simulink model "trim_homework태원"  (R2023b)
settings: Solver=VariableStepAuto  StartTime=0.0  StopTime=200  RelTol=1e-3
model workspace (MAT data in the model file):
  op_trim1 = opcond.OperatingReport
  op_trim1.Outputs_ = opcond.OutputReport
  op_trim1.Outputs_.yspec_ = 23
  op_trim1.Outputs_.Block_ = 'trim_homework/Va'
  op_trim1.Outputs_.PortWidth_ = 1
  op_trim1.Outputs_.PortNumber_ = NaN
  op_trim1.Outputs_.y_ = 23
  op_trim1.Outputs_.Known_ = 1
  op_trim1.Outputs_.Min_ = -Inf
  op_trim1.Outputs_.Max_ = Inf
  op_trim1.TerminationString_ = '동작점 사양이 성공적으로 충족되었습니다.'
  op_trim1.OptimizationOutput_.iterations = 4
  op_trim1.OptimizationOutput_.funcCount = 67
  op_trim1.OptimizationOutput_.lssteplength = 1
  op_trim1.OptimizationOutput_.stepsize = 1.37227351892e-10
  op_trim1.OptimizationOutput_.algorithm = 'active-set'
  op_trim1.OptimizationOutput_.firstorderopt = 0
  op_trim1.OptimizationOutput_.constrviolation = 8.72514182054e-12
  op_trim1.OptimizationOutput_.message = '제약 조건을 충족하는 국소 최솟값을 찾았습니다.
    | 
    | 목적 함수가 최적성 허용오차의 값 이내에서 실현 가능한 방향에서 감소하지 않고 
    | 제약 조건이 제약 조건 허용오차의 값 이내에서 충족되기 때문에 
    | 최적화가 완료되었습니다.
    | 
    | <중지 기준 세부 정보>
    | 
    | 최적화가 완료됨: 1차 최적성 측정값 0.000000e+00이(가)
    | options.OptimalityTolerance = 1.000000e-06보다 작고 최대 제약 조건 위반
    | 8.725142e-12이(가) options.ConstraintTolerance = 1.000000e-06보다 작습니다.'
  op_trim1.OptimizationOutput_.bestfeasible.x = [22.9488032673; 3.41196938771e-08; 1.53376288852; 1.51318063862e-09; 0.0667348663763; -1.38255798073e-09; 1.08686704389e-15; -3.74282177879e-15; 1.13331068217e-24; 4.09052789101e-22; 7.74880795459e-26; 1.11476618756e-09; -0.171064175627; 1.39174657063e-09; 11.2753696029]
  op_trim1.OptimizationOutput_.bestfeasible.fval = 0
  op_trim1.OptimizationOutput_.bestfeasible.constrviolation = 8.72514182054e-12
  op_trim1.OptimizationOutput_.bestfeasible.firstorderopt = 0
  op_trim1.OptimizationOutput_.progress = {'<font face="monospaced"; size=3><BR>', '원하는 dx/dt=0, x(k+1)-x(k)=0, y=ydes 전체에 대해 해를 구하기 위해 최적화합니다.<BR>', ' <BR>', '(최대 오차) 블록<BR>', ' ---------------------------------------------------------<BR>', '(5.95306e+00) trim_homework/6DOF (Euler Angles)/ub,vb,wb<BR>', '(3.93818e-01) trim_homework/6DOF (Euler Angles)/ub,vb,wb<BR>', '(2.71037e-05) trim_homework/6DOF (Euler Angles)/ub,vb,wb<BR>', '(8.72514e-12) trim_homework/6DOF (Euler Angles)/ub,vb,wb<BR>', '(8.72514e-12) trim_homework/6DOF (Euler Angles)/ub,vb,wb<BR>', ' <BR>', '동작점 사양이 성공적으로 충족되었습니다.<BR>'}
  op_trim1.Model_ = 'trim_homework'
  op_trim1.States_(1) = opcond.StateReport
  op_trim1.States_(1).dx_ = [1.13848957052e-24; 4.09052789101e-22; 7.76615688898e-26]
  op_trim1.States_(1).Nx_ = 3
  op_trim1.States_(1).Block_ = 'trim_homework/6DOF (Euler Angles)/Calculate DCM &
    | Euler Angles/phi
    | theta
    | psi'
  op_trim1.States_(1).x_ = [1.51318063862e-09; 0.0667348663763; -1.38255798073e-09]
  op_trim1.States_(1).SteadyState_ = [1; 1; 1]
  op_trim1.States_(1).dxMin_ = [-Inf; -Inf; -Inf]
  op_trim1.States_(1).dxMax_ = [Inf; Inf; Inf]
  op_trim1.States_(1).Known_ = [0; 0; 0]
  op_trim1.States_(1).Min_ = [-Inf; -Inf; -Inf]
  op_trim1.States_(1).Max_ = [Inf; Inf; Inf]
  op_trim1.States_(2) = opcond.StateReport
  op_trim1.States_(2).dx_ = [8.46060064603e-19; 3.2482900909e-13; -1.72544390739e-19]
  op_trim1.States_(2).Nx_ = 3
  op_trim1.States_(2).Block_ = 'trim_homework/6DOF (Euler Angles)/p,q,r '
  op_trim1.States_(2).x_ = [1.13331068217e-24; 4.09052789101e-22; 7.74880795459e-26]
  op_trim1.States_(2).SteadyState_ = [1; 1; 1]
  op_trim1.States_(2).dxMin_ = [-Inf; -Inf; -Inf]
  op_trim1.States_(2).dxMax_ = [Inf; Inf; Inf]
  op_trim1.States_(2).Known_ = [0; 0; 0]
  op_trim1.States_(2).Min_ = [-Inf; -Inf; -Inf]
  op_trim1.States_(2).Max_ = [Inf; Inf; Inf]
  op_trim1.States_(3) = opcond.StateReport
  op_trim1.States_(3).dx_ = [8.72514182054e-12; 4.3787508586e-19; -2.2478987429e-13]
  op_trim1.States_(3).Nx_ = 3
  op_trim1.States_(3).Block_ = 'trim_homework/6DOF (Euler Angles)/ub,vb,wb'
  op_trim1.States_(3).x_ = [22.9488032673; 3.41196938771e-08; 1.53376288852]
  op_trim1.States_(3).SteadyState_ = [1; 1; 1]
  op_trim1.States_(3).dxMin_ = [-Inf; -Inf; -Inf]
  op_trim1.States_(3).dxMax_ = [Inf; Inf; Inf]
  op_trim1.States_(3).Known_ = [0; 0; 0]
  op_trim1.States_(3).Min_ = [-Inf; -Inf; -Inf]
  op_trim1.States_(3).Max_ = [Inf; Inf; Inf]
  op_trim1.States_(4) = opcond.StateReport
  op_trim1.States_(4).dx_ = [23; 1.31654190371e-17; 4.10782519111e-14]
  op_trim1.States_(4).Nx_ = 3
  op_trim1.States_(4).Block_ = 'trim_homework/6DOF (Euler Angles)/xe,ye,ze'
  op_trim1.States_(4).x_ = [1.08686704389e-15; -3.74282177879e-15; -200]
  op_trim1.States_(4).SteadyState_ = [0; 1; 1]
  op_trim1.States_(4).dxMin_ = [-Inf; -Inf; -Inf]
  op_trim1.States_(4).dxMax_ = [Inf; Inf; Inf]
  op_trim1.States_(4).Known_ = [0; 0; 1]
  op_trim1.States_(4).Min_ = [-Inf; -Inf; -Inf]
  op_trim1.States_(4).Max_ = [Inf; Inf; Inf]
  op_trim1.Inputs_(1) = opcond.InputReport
  op_trim1.Inputs_(1).Block_ = 'trim_homework/AIL'
  op_trim1.Inputs_(1).PortWidth_ = 1
  op_trim1.Inputs_(1).PortDimensions_ = [1 1]
  op_trim1.Inputs_(1).u_ = 1.11476618756e-09
  op_trim1.Inputs_(1).Known_ = 0
  op_trim1.Inputs_(1).Min_ = -Inf
  op_trim1.Inputs_(1).Max_ = Inf
  op_trim1.Inputs_(2) = opcond.InputReport
  op_trim1.Inputs_(2).Block_ = 'trim_homework/ELE'
  op_trim1.Inputs_(2).PortWidth_ = 1
  op_trim1.Inputs_(2).PortDimensions_ = [1 1]
  op_trim1.Inputs_(2).u_ = -0.171064175627
  op_trim1.Inputs_(2).Known_ = 0
  op_trim1.Inputs_(2).Min_ = -Inf
  op_trim1.Inputs_(2).Max_ = Inf
  op_trim1.Inputs_(3) = opcond.InputReport
  op_trim1.Inputs_(3).Block_ = 'trim_homework/RUD'
  op_trim1.Inputs_(3).PortWidth_ = 1
  op_trim1.Inputs_(3).PortDimensions_ = [1 1]
  op_trim1.Inputs_(3).u_ = 1.39174657063e-09
  op_trim1.Inputs_(3).Known_ = 0
  op_trim1.Inputs_(3).Min_ = -Inf
  op_trim1.Inputs_(3).Max_ = Inf
  op_trim1.Inputs_(4) = opcond.InputReport
  op_trim1.Inputs_(4).Block_ = 'trim_homework/Thro'
  op_trim1.Inputs_(4).PortWidth_ = 1
  op_trim1.Inputs_(4).PortDimensions_ = [1 1]
  op_trim1.Inputs_(4).u_ = 11.2753696029
  op_trim1.Inputs_(4).Known_ = 0
  op_trim1.Inputs_(4).Min_ = -Inf
  op_trim1.Inputs_(4).Max_ = Inf
  op_trim2 = opcond.OperatingReport
  op_trim2.Outputs_ = opcond.OutputReport
  op_trim2.Outputs_.yspec_ = 23
  op_trim2.Outputs_.Block_ = 'trim_homework/Va'
  op_trim2.Outputs_.PortWidth_ = 1
  op_trim2.Outputs_.PortNumber_ = NaN
  op_trim2.Outputs_.y_ = 1
  op_trim2.Outputs_.Known_ = 1
  op_trim2.Outputs_.Min_ = -Inf
  op_trim2.Outputs_.Max_ = Inf
  op_trim2.TerminationString_ = '모든 제약 조건을 충족하는 해를 찾을 수 없습니다. 실현 가능한 해를 찾으려면 제약 조건을 완화하십시오.'
  op_trim2.OptimizationOutput_.iterations = 1
  op_trim2.OptimizationOutput_.funcCount = 25
  op_trim2.OptimizationOutput_.lssteplength = 1
  op_trim2.OptimizationOutput_.stepsize = 0
  op_trim2.OptimizationOutput_.algorithm = 'active-set'
  op_trim2.OptimizationOutput_.firstorderopt = []
  op_trim2.OptimizationOutput_.constrviolation = 22
  op_trim2.OptimizationOutput_.message = '실현불가능점으로 수렴되었습니다.
    | 
    | 현재 탐색 방향의 크기가 스텝 크기 허용오차 값의 두 배보다 
    | 작지만 제약 조건이 제약 조건 허용오차의 값 이내에서 
    | 충족되지 않기 때문에 fmincon이(가) 중지되었습니다.
    | 
    | <중지 기준 세부 정보>
    | 
    | 현재 탐색 방향의 노름 0.000000e+00이(가) 2*options.StepTolerance = 1.000000e-06보다
    | 작지만 최대 제약 조건 위반 2.200000e+01이(가) options.ConstraintTolerance = 1.000000e-06을(를)
    | 초과하기 때문에 최적화가 중지되었습니다.'
  op_trim2.OptimizationOutput_.bestfeasible = []
  op_trim2.OptimizationOutput_.progress = {'<font face="monospaced"; size=3><BR>', '원하는 dx/dt=0, x(k+1)-x(k)=0, y=ydes 전체에 대해 해를 구하기 위해 최적화합니다.<BR>', ' <BR>', '(최대 오차) 블록<BR>', ' ---------------------------------------------------------<BR>', '(2.20000e+01) trim_homework/Va<BR>', '(2.20000e+01) trim_homework/Va<BR>', ' <BR>', '모든 제약 조건을 충족하는 해를 찾을 수 없습니다. 실현 가능한 해를 찾으려면 제약 조건을 완화하십시오.<BR>'}
  op_trim2.Model_ = 'trim_homework'
  op_trim2.States_(1) = opcond.StateReport
  op_trim2.States_(1).dx_ = [0; 0; 0]
  op_trim2.States_(1).Nx_ = 3
  op_trim2.States_(1).Block_ = 'trim_homework/6DOF (Quaternion)/Calculate DCM &
    | Euler Angles/phi
    | theta
    | psi'
  op_trim2.States_(1).x_ = [0; 0; 0]
  op_trim2.States_(1).SteadyState_ = [1; 1; 1]
  op_trim2.States_(1).dxMin_ = [-Inf; -Inf; -Inf]
  op_trim2.States_(1).dxMax_ = [Inf; Inf; Inf]
  op_trim2.States_(1).Known_ = [0; 0; 0]
  op_trim2.States_(1).Min_ = [-Inf; -Inf; -Inf]
  op_trim2.States_(1).Max_ = [Inf; Inf; Inf]
  op_trim2.States_(2) = opcond.StateReport
  op_trim2.States_(2).dx_ = [0; 0.000788031277533; 0]
  op_trim2.States_(2).Nx_ = 3
  op_trim2.States_(2).Block_ = 'trim_homework/6DOF (Quaternion)/p,q,r '
  op_trim2.States_(2).x_ = [0; 0; 0]
  op_trim2.States_(2).SteadyState_ = [1; 1; 1]
  op_trim2.States_(2).dxMin_ = [-Inf; -Inf; -Inf]
  op_trim2.States_(2).dxMax_ = [Inf; Inf; Inf]
  op_trim2.States_(2).Known_ = [0; 0; 0]
  op_trim2.States_(2).Min_ = [-Inf; -Inf; -Inf]
  op_trim2.States_(2).Max_ = [Inf; Inf; Inf]
  op_trim2.States_(3) = opcond.StateReport
  op_trim2.States_(3).dx_ = [-0.0013631; 0; 9.802709]
  op_trim2.States_(3).Nx_ = 3
  op_trim2.States_(3).Block_ = 'trim_homework/6DOF (Quaternion)/ub,vb,wb'
  op_trim2.States_(3).x_ = [1; 0; 0]
  op_trim2.States_(3).SteadyState_ = [1; 1; 1]
  op_trim2.States_(3).dxMin_ = [-Inf; -Inf; -Inf]
  op_trim2.States_(3).dxMax_ = [Inf; Inf; Inf]
  op_trim2.States_(3).Known_ = [0; 0; 0]
  op_trim2.States_(3).Min_ = [-Inf; -Inf; -Inf]
  op_trim2.States_(3).Max_ = [Inf; Inf; Inf]
  op_trim2.States_(4) = opcond.StateReport
  op_trim2.States_(4).dx_ = [1; 0; 0]
  op_trim2.States_(4).Nx_ = 3
  op_trim2.States_(4).Block_ = 'trim_homework/6DOF (Quaternion)/xe,ye,ze'
  op_trim2.States_(4).x_ = [0; 0; -200]
  op_trim2.States_(4).SteadyState_ = [0; 1; 1]
  op_trim2.States_(4).dxMin_ = [-Inf; -Inf; -Inf]
  op_trim2.States_(4).dxMax_ = [Inf; Inf; Inf]
  op_trim2.States_(4).Known_ = [0; 0; 1]
  op_trim2.States_(4).Min_ = [-Inf; -Inf; -Inf]
  op_trim2.States_(4).Max_ = [Inf; Inf; Inf]
  op_trim2.States_(5) = opcond.StateReport
  op_trim2.States_(5).dx_ = [0; 0; 0]
  op_trim2.States_(5).Nx_ = 3
  op_trim2.States_(5).Block_ = 'trim_homework/6DOF (Quaternion)1/Calculate DCM &
    | Euler Angles/phi
    | theta
    | psi'
  op_trim2.States_(5).x_ = [0; 0; 0]
  op_trim2.States_(5).SteadyState_ = [1; 1; 1]
  op_trim2.States_(5).dxMin_ = [-Inf; -Inf; -Inf]
  op_trim2.States_(5).dxMax_ = [Inf; Inf; Inf]
  op_trim2.States_(5).Known_ = [0; 0; 0]
  op_trim2.States_(5).Min_ = [-Inf; -Inf; -Inf]
  op_trim2.States_(5).Max_ = [Inf; Inf; Inf]
  op_trim2.States_(6) = opcond.StateReport
  op_trim2.States_(6).dx_ = [0; 0; 0]
  op_trim2.States_(6).Nx_ = 3
  op_trim2.States_(6).Block_ = 'trim_homework/6DOF (Quaternion)1/p,q,r '
  op_trim2.States_(6).x_ = [0; 0; 0]
  op_trim2.States_(6).SteadyState_ = [1; 1; 1]
  op_trim2.States_(6).dxMin_ = [-Inf; -Inf; -Inf]
  op_trim2.States_(6).dxMax_ = [Inf; Inf; Inf]
  op_trim2.States_(6).Known_ = [0; 0; 0]
  op_trim2.States_(6).Min_ = [-Inf; -Inf; -Inf]
  op_trim2.States_(6).Max_ = [Inf; Inf; Inf]
  op_trim2.States_(7) = opcond.StateReport
  op_trim2.States_(7).dx_ = [0; 0; 0]
  op_trim2.States_(7).Nx_ = 3
  op_trim2.States_(7).Block_ = 'trim_homework/6DOF (Quaternion)1/ub,vb,wb'
  op_trim2.States_(7).x_ = [0; 0; 0]
  op_trim2.States_(7).SteadyState_ = [1; 1; 1]
  op_trim2.States_(7).dxMin_ = [-Inf; -Inf; -Inf]
  op_trim2.States_(7).dxMax_ = [Inf; Inf; Inf]
  op_trim2.States_(7).Known_ = [0; 0; 0]
  op_trim2.States_(7).Min_ = [-Inf; -Inf; -Inf]
  op_trim2.States_(7).Max_ = [Inf; Inf; Inf]
  op_trim2.States_(8) = opcond.StateReport
  op_trim2.States_(8).dx_ = [0; 0; 0]
  op_trim2.States_(8).Nx_ = 3
  op_trim2.States_(8).Block_ = 'trim_homework/6DOF (Quaternion)1/xe,ye,ze'
  op_trim2.States_(8).x_ = [0; 0; 0]
  op_trim2.States_(8).SteadyState_ = [1; 1; 1]
  op_trim2.States_(8).dxMin_ = [-Inf; -Inf; -Inf]
  op_trim2.States_(8).dxMax_ = [Inf; Inf; Inf]
  op_trim2.States_(8).Known_ = [0; 0; 0]
  op_trim2.States_(8).Min_ = [-Inf; -Inf; -Inf]
  op_trim2.States_(8).Max_ = [Inf; Inf; Inf]
  op_trim2.Inputs_ = opcond.InputReport
  op_trim2.Inputs_.Block_ = 'trim_homework/ELE_Trim'
  op_trim2.Inputs_.PortWidth_ = 1
  op_trim2.Inputs_.PortDimensions_ = [1 1]
  op_trim2.Inputs_.Known_ = 0
  op_trim2.Inputs_.Min_ = -Inf
  op_trim2.Inputs_.Max_ = Inf
undefined symbols (not defined in the file or in its folder): deg, rad, s
libraries: aerolibconvert2 x2, shared6dof x1, aerolibasang x1
settings Model: Creator=UASG  LastModifiedBy=UASG
settings DataIOCC: ExternalInput=getinputstruct(op_trim1)  InitialState=getstatestruct(op_trim1)  LoadExternalInput=on  LoadInitialState=on

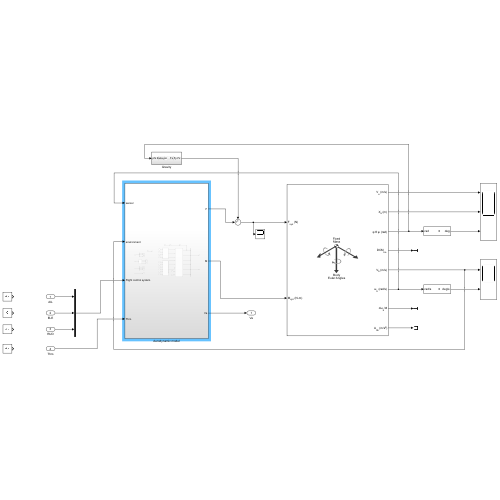
[thumbnail: Simulink's stored preview of the top-level diagram]
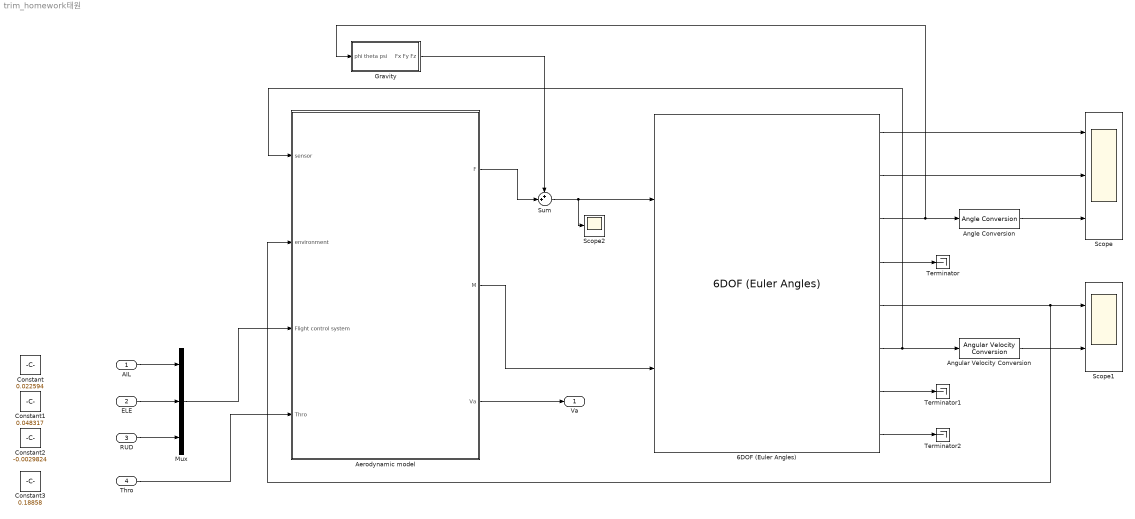
== system trim_homework태원 ==
  AIL : Inport
  ELE : Inport  Port=2
  RUD : Inport  Port=3
  Thro : Inport  Port=4
  6DOF (Euler Angles) : shared6dof/6DOF (Euler Angles)  units=Metric (MKS)  mtype=Fixed  rep=Euler Angles  xme_0=[0 0 -200]  Vm_0=[1 0 0]  eul_0=[0 0 0]  pm_0=[0 0 0]  mass_0=11  mass_e=0.5  mass_f=2.0  inertia=[0.824 0 -0.120; 0 1.135 0; -0.120 0 1.759]  inertia_e=eye(3)  inertia_f=2*eye(3)  k_quat=1.0  vre_flag=on  abi_flag=off  aMode=0  xme_statename=''  Vm_statename=''  eul_statename=''  quat_statename=''  pm_statename=''  mass_statename=''
  Aerodynamic model : Subsystem
  Angle Conversion : aerolibconvert2/Angle Conversion  IU=rad  OU=deg
  Angular Velocity Conversion : aerolibconvert2/Angular Velocity Conversion  IU=rad/s  OU=deg/s
  Constant : Constant  Value=0.022594
  Constant1 : Constant  Value=0.048317
  Constant2 : Constant  Value=-0.0029824
  Constant3 : Constant  Value=0.18858
  Gravity : Subsystem
  Mux : Mux  Inputs=3
  Scope : Scope  NumInputPorts=3
  Scope1 : Scope  NumInputPorts=2
  Scope2 : Scope
  Sum : Sum  Inputs=++|
  Terminator : Terminator
  Terminator1 : Terminator
  Terminator2 : Terminator
  Va : Outport
  wires:
  6DOF (Euler Angles)/6 -> Angular Velocity Conversion/1, Aerodynamic model/1(sensor)
  6DOF (Euler Angles)/5 -> Aerodynamic model/2(environment), Scope1/1
  Mux/1 -> Aerodynamic model/3(Flight control system)
  6DOF (Euler Angles)/1 -> Scope/1
  6DOF (Euler Angles)/2 -> Scope/2
  6DOF (Euler Angles)/3 -> Gravity/1(phi theta psi), Angle Conversion/1
  Angular Velocity Conversion/1 -> Scope1/2
  Angle Conversion/1 -> Scope/3
  6DOF (Euler Angles)/4 -> Terminator/1
  6DOF (Euler Angles)/7 -> Terminator1/1
  6DOF (Euler Angles)/8 -> Terminator2/1
  Aerodynamic model/2(M) -> 6DOF (Euler Angles)/2
  Aerodynamic model/1(F) -> Sum/2
  Gravity/1(Fx Fy Fz) -> Sum/1
  Aerodynamic model/3(Va) -> Va/1
  Sum/1 -> Scope2/1, 6DOF (Euler Angles)/1
  AIL/1 -> Mux/1
  ELE/1 -> Mux/2
  RUD/1 -> Mux/3
  Thro/1 -> Aerodynamic model/4(Thro)

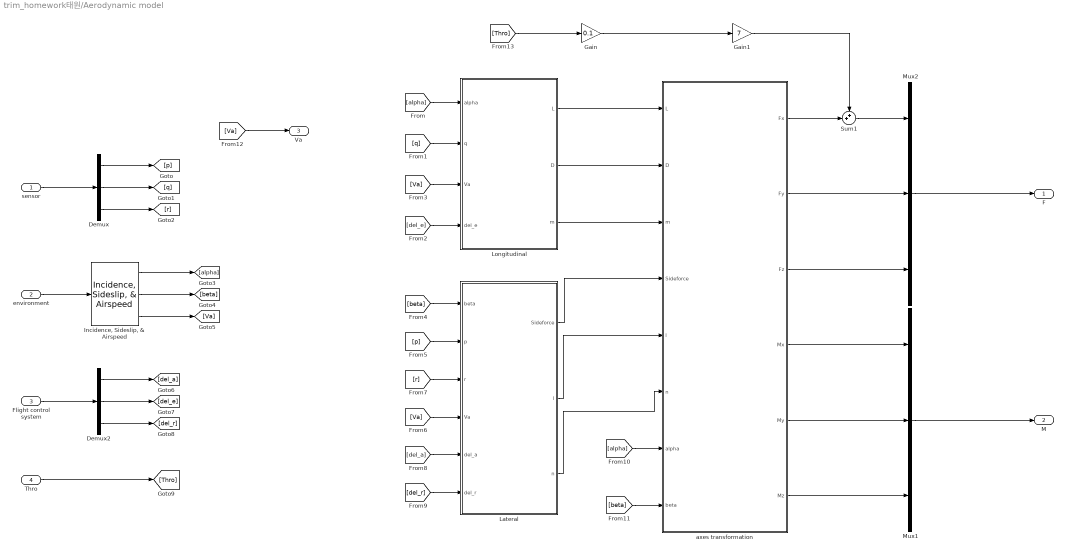
== system trim_homework태원/Aerodynamic model ==
  sensor : Inport
  environment : Inport  Port=2
  Flight control system : Inport  Port=3
  Thro : Inport  Port=4
  Demux : Demux  Outputs=3
  Demux2 : Demux  Outputs=3
  Gain : Gain  Gain=0.1
  Gain1 : Gain  Gain=7
  "Incidence, Sideslip, & Airspeed" : aerolibasang/Incidence, Sideslip, & Airspeed
  Lateral : MATLAB Function  TreatAsAtomicUnit=on
  Longitudinal : MATLAB Function  TreatAsAtomicUnit=on
  Mux1 : Mux  Inputs=3
  Mux2 : Mux  Inputs=3
  Sum1 : Sum  Inputs=++|
  axes transformation : Subsystem
  F : Outport
  M : Outport  Port=2
  Va : Outport  Port=3
  wires:
  [alpha] -> Longitudinal/1(alpha)
  [q] -> Longitudinal/2(q)
  [Va] -> Longitudinal/3(Va)
  [del_e] -> Longitudinal/4(del_e)
  [beta] -> Lateral/1(beta)
  [p] -> Lateral/2(p)
  [r] -> Lateral/3(r)
  [Va] -> Lateral/4(Va)
  [del_a] -> Lateral/5(del_a)
  [del_r] -> Lateral/6(del_r)
  Longitudinal/1(L) -> axes transformation/1(L)
  Longitudinal/2(D) -> axes transformation/2(D)
  Longitudinal/3(m) -> axes transformation/3(m)
  Lateral/1(Sideforce) -> axes transformation/4(Sideforce)
  Lateral/2(l) -> axes transformation/5(l)
  Lateral/3(n) -> axes transformation/6(n)
  [alpha] -> axes transformation/7(alpha)
  [beta] -> axes transformation/8(beta)
  sensor/1 -> Demux/1
  Demux/1 -> [p]
  Demux/2 -> [q]
  Demux/3 -> [r]
  "Incidence, Sideslip, & Airspeed"/1 -> [alpha]
  "Incidence, Sideslip, & Airspeed"/2 -> [beta]
  "Incidence, Sideslip, & Airspeed"/3 -> [Va]
  Demux2/2 -> [del_e]
  Demux2/3 -> [del_r]
  Demux2/1 -> [del_a]
  Flight control system/1 -> Demux2/1
  axes transformation/5(My) -> Mux1/2
  axes transformation/4(Mx) -> Mux1/1
  axes transformation/6(Mz) -> Mux1/3
  axes transformation/2(Fy) -> Mux2/2
  axes transformation/3(Fz) -> Mux2/3
  Mux1/1 -> M/1
  environment/1 -> "Incidence, Sideslip, & Airspeed"/1
  [Va] -> Va/1
  Thro/1 -> [Thro]
  [Thro] -> Gain/1
  Gain/1 -> Gain1/1
  Mux2/1 -> F/1
  axes transformation/1(Fx) -> Sum1/2
  Sum1/1 -> Mux2/1
  Gain1/1 -> Sum1/1

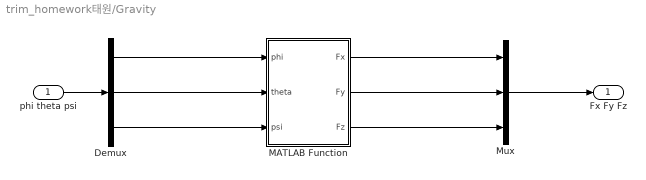
== system trim_homework태원/Gravity ==
  phi theta psi : Inport
  Demux : Demux  Outputs=3
  MATLAB Function : MATLAB Function  TreatAsAtomicUnit=on
  Mux : Mux  Inputs=3
  Fx Fy Fz : Outport
  wires:
  phi theta psi/1 -> Demux/1
  Demux/1 -> MATLAB Function/1(phi)
  Demux/2 -> MATLAB Function/2(theta)
  Demux/3 -> MATLAB Function/3(psi)
  MATLAB Function/2(Fy) -> Mux/2
  MATLAB Function/1(Fx) -> Mux/1
  MATLAB Function/3(Fz) -> Mux/3
  Mux/1 -> Fx Fy Fz/1

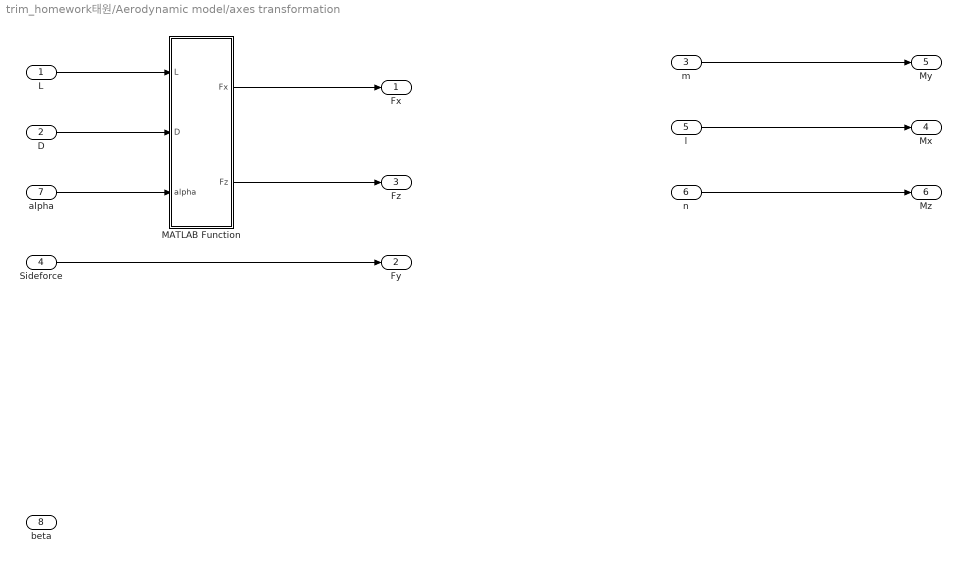
== system trim_homework태원/Aerodynamic model/axes transformation ==
  L : Inport
  D : Inport  Port=2
  m : Inport  Port=3
  Sideforce : Inport  Port=4
  l : Inport  Port=5
  n : Inport  Port=6
  alpha : Inport  Port=7
  beta : Inport  Port=8
  MATLAB Function : MATLAB Function  TreatAsAtomicUnit=on
  Fx : Outport
  Fy : Outport  Port=2
  Fz : Outport  Port=3
  Mx : Outport  Port=4
  My : Outport  Port=5
  Mz : Outport  Port=6
  wires:
  l/1 -> Mx/1
  m/1 -> My/1
  n/1 -> Mz/1
  Sideforce/1 -> Fy/1
  L/1 -> MATLAB Function/1(L)
  D/1 -> MATLAB Function/2(D)
  alpha/1 -> MATLAB Function/3(alpha)
  MATLAB Function/2(Fz) -> Fz/1
  MATLAB Function/1(Fx) -> Fx/1

== matlab function trim_homework태원/Aerodynamic model/Lateral ==
  data: beta input; Sideforce output; p input; r input; Va input; l output; n output; del_a input; del_r input
function [Sideforce, l, n] = fnc(beta, p, r, Va, del_a, del_r)

%Lateral Aerodynamics

%% Coefficients
m = 11.0; %kg
Ix = 0.824; %kg*m^2
Iy = 1.135; %kg*m^2
Iz = 1.759; %kg*m^2
Ixz = 0.120; %kg*m^2
S = 0.55; %m^2
b = 2.9; %m
c = 0.19; %m
rho = 1.268; %kg/m^3
e = 0.9;
CL0 = 0.23;
CD0 = 0.043;
Cm0 = 0.0135;
CLalpha = 5.61;
CDalpha = 0.030;
Cmalpha = -2.74;
CLq = 7.95;
CDq = 0;
Cmq = -38.21;
CLdel_e = 0.13;
CDdel_e = 0.0135;
Cmdel_e = -0.99;
M = 50;
alpha0 = 0.47;
epsilon = 0.16;
CDp = 0;
CY0 = 0;
Cl0 = 0;
Cn0 = 0;
CYbeta = -0.83;
Clbeta = -0.13;
Cnbeta = 0.073;
CYp = 0;
Clp = -0.51;
Cnp = -0.069;
CYr = 0;
Clr = 0.25;
Cnr = -0.095;
CYdel_a = 0.075;
Cldel_a = 0.17;
Cndel_a = -0.011;
CYdel_r = 0.19;
Cldel_r = 0.0024;
Cndel_r = -0.069;

%% Aerodynamic forces and moments(Longitudinal Aerodynamics)
Sideforce = 0.5*rho*(Va^2)*S*(CY0+CYbeta*beta+CYp*b/2/Va*p+CYr*b/2/Va*r+CYdel_a*del_a+CYdel_r*del_r);
l = 0.5*rho*(Va^2)*S*b*(Cl0+Clbeta*beta+Clp*b/2/Va*p+Clr*b/2/Va*r+Cldel_a*del_a+Cldel_r*del_r);
n = 0.5*rho*(Va^2)*S*b*(Cn0+Cnbeta*beta+Cnp*b/2/Va*p+Cnr*b/2/Va*r+Cndel_a*del_a+Cndel_r*del_r);

== matlab function trim_homework태원/Aerodynamic model/Longitudinal ==
  data: alpha input; L output; q input; Va input; del_e input; D output; m output
function [L,D,m] = fnc(alpha, q, Va, del_e)

%Longitudinal Aerodynamics

%% Coefficients
m = 11.0; %kg
Ix = 0.824; %kg*m^2
Iy = 1.135; %kg*m^2
Iz = 1.759; %kg*m^2
Ixz = 0.120; %kg*m^2
S = 0.55; %m^2
b = 2.9; %m
c = 0.19; %m
rho = 1.268; %kg/m^3
e = 0.9;
CL0 = 0.23;
CD0 = 0.043;
Cm0 = 0.0135;
CLalpha = 5.61;
CDalpha = 0.030;
Cmalpha = -2.74;
CLq = 7.95;
CDq = 0;
Cmq = -38.21;
CLdel_e = 0.13;
CDdel_e = 0.0135;
Cmdel_e = -0.99;
M = 50;
alpha0 = 0.47;
epsilon = 0.16;
CDp = 0;
CY0 = 0;
Cl0 = 0;
Cn0 = 0;
CYbeta = -0.83;
Clbeta = -0.13;
Cnbeta = 0.073;
CYp = 0;
Clp = -0.51;
Cnp = -0.069;
CYr = 0;
Clr = 0.25;
Cnr = -0.095;
CYdel_a = 0.075;
Cldel_a = 0.17;
Cndel_a = -0.011;
CYdel_r = 0.19;
Cldel_r = 0.0024;
Cndel_r = -0.069;

%% Aerodynamic forces and moments(Longitudinal Aerodynamics)
L = 0.5*rho*Va^2*S*(CL0+CLalpha*alpha+CLq*c/2/Va*q+CLdel_e*del_e);
D = 0.5*rho*Va^2*S*(CD0+CDalpha*alpha+CDq*c/2/Va*q+CDdel_e*del_e);
m = 0.5*rho*Va^2*S*c*(Cm0+Cmalpha*alpha+Cmq*c/2/Va*q+Cmdel_e*del_e);

== matlab function trim_homework태원/Aerodynamic model/axes transformation/MATLAB Function ==
  data: L input; D input; alpha input; Fx output; Fz output
function [Fx, Fz] = fcn(L, D, alpha)

Fx = -cos(alpha)*D + sin(alpha)*L;
Fz = -sin(alpha)*D - cos(alpha)*L;

== matlab function trim_homework태원/Gravity/MATLAB Function ==
  data: phi input; theta input; psi input; Fx output; Fy output; Fz output
function [Fx, Fy, Fz] = fcn(phi, theta, psi)

m = 11; %kg
g = 9.81; %m/s^2

Fx = -m*g*sin(theta);
Fy = m*g*cos(theta)*sin(phi);
Fz = m*g*cos(theta)*cos(phi);
